simulink model "rotating_pendulum_3states_simulink"  (R2020b)
settings: Solver=FixedStepAuto  StartTime=0.0  StopTime=40  FixedStep=h  RelTol=1e-3  EnableMultiTasking=on
values from neighbouring files (symbols this model uses):
  adingain = [adingain 1 1 1 1 1]    [hwinit.m]
  adinoffs = [adinoffs 0 0 0 0 0]    [hwinit.m]
  daoutgain = 1*[-6]    [hwinit.m]
  daoutoffs = [0.00]    [hwinit.m]
  h = 0.01    [Linearization_4state.m]    (also in hwinit.m = 0.001; rotpentest.m = fugiboard('Open', 'pendulum1'))
  K = model.Km    [Linearization_4state.m]    (also in Model_derivation.m = K_trans + K_rot; Model_derivation_4_states.m = K_trans + K_rot; dc_motor_control.m = dlqr(dt_sys_zoh.A, dt_sys_zoh.B, Q_lqr, R_lqr); identification_dc_motor.m = -0.05)
  K_ff = 1/dcgain_sys    [dc_motor_control.m]    (also in rotating_pendulum_3states.m; rotating_pendulum_4states.m)
  R_kf = 1 * diag([1, 10, 1, 10])    [dc_motor_control.m]    (also in rotating_pendulum_3states.m = 50 * diag([1, 1, 10]); rotating_pendulum_4states.m = diag([7.5740e-06, 0.1526, 1.4489e-05, 0.2930]))
undefined symbols (not defined in the file or in its folder): Discrete, Time
libraries: simulink x3, ctrlSharedLib x1
settings Model: Creator=rbabuska  LastModifiedBy=dlooman
settings DataIOCC: LimitDataPoints=on  SaveFormat=Array  ReturnWorkspaceOutputs=off  SignalLoggingName=sigsOut
settings OptimizationCC: BooleanDataType=off  ExpressionDepthLimit=2147483647  InitFltsAndDblsToZero=on  LifeSpan=inf
settings DebuggingCC: SaveWithParameterizedLinksMsg=none  SignalResolutionControl=TryResolveAllWithWarning  MultiTaskDSMMsg=warning  MultiTaskCondExecSysMsg=none  AllowSymbolicDim=off  StateNameClashWarn=warning  SFUnexpectedBacktrackingDiag=warning  SFNoUnconditionalDefaultTransitionDiag=warning  SFExecutionAtInitializationDiag=none  ArithmeticOperatorsInVariantConditions=warning
settings HardwareCC: ProdBitPerPointer=32  ProdBitPerSizeT=32  ProdBitPerPtrDiffT=32  ProdLargestAtomicFloat=None  ProdIntDivRoundTo=Undefined  ProdEndianess=Unspecified  ProdWordSize=32  ProdHWDeviceType=32-bit Generic  TargetUnknown=on
settings ModelReferenceCC: PropagateSignalLabelsOutOfModel=off
settings SFSimCC: SimUseLocalCustomCode=off  CustomCodeUndefinedFunction=UseInterfaceOnly
settings RTWCC: RTWUseLocalCustomCode=off
settings CodeAppCC: StateflowObjectComments=on
settings GRTTargetCC: TargetFcnLib=ansi_tfl_tmw.mat  TargetLangStandard=C89/C90 (ANSI)  CombineOutputUpdateFcns=off  GRTInterface=on
settings ConfigComp: CovMetricSettings=dw  CovSaveCumulativeToWorkspaceVar=on  CovSaveSingleToWorkspaceVar=on  CovExternalEMLEnable=off

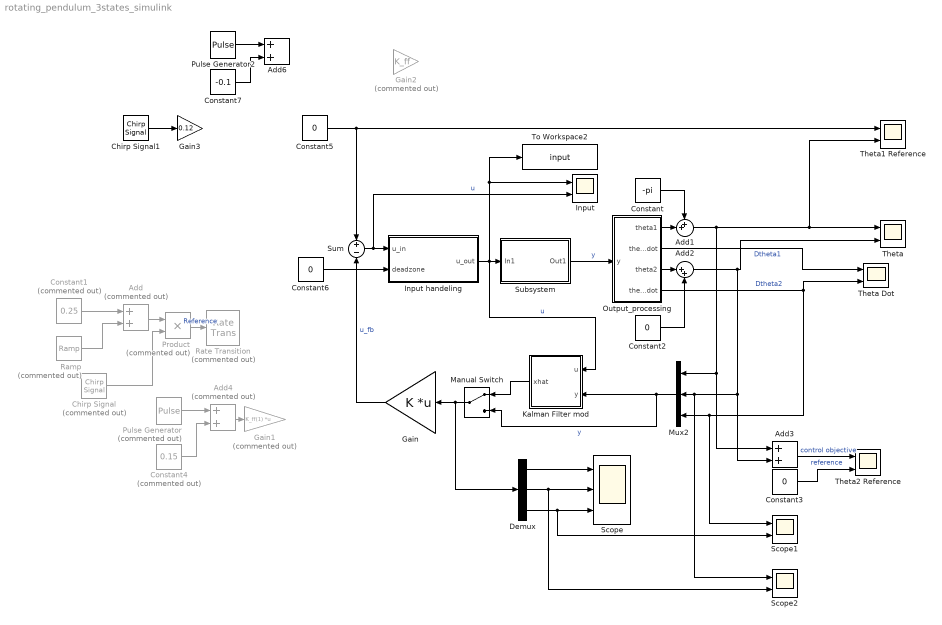
== system rotating_pendulum_3states_simulink ==
  Add : Sum  Commented=on
  Add1 : Sum  Inputs=++|
  Add2 : Sum  Inputs=|++
  Add3 : Sum
  Add4 : Sum  Commented=on
  Add6 : Sum
  Chirp Signal : simulink/Sources/Chirp Signal  Commented=on  f1=3  T=20  f2=1
  Chirp Signal1 : simulink/Sources/Chirp Signal  f1=0.1  T=20  f2=2.5
  Constant : Constant  Value=-pi
  Constant1 : Constant  Commented=on  Value=0.25  SampleTime=h
  Constant{2..3,5..6} (4 alike) : Constant  Value=0
  Constant4 : Constant  Commented=on  Value=0.15
  Constant7 : Constant  Value=-0.1
  Demux : Demux  Outputs=3
  Gain : Gain  Gain=K  Multiplication=Matrix(K*u)
  Gain1 : Gain  Commented=on  Gain=K_ff(1)  Multiplication=Matrix(K*u)
  Gain2 : Gain  Commented=on  Gain=K_ff
  Gain3 : Gain  Gain=0.12
  Input : Scope  NumInputPorts=2
  Input handeling : MATLAB Function  TreatAsAtomicUnit=on
  Kalman Filter mod : Subsystem
  Manual Switch : ManualSwitch
  Mux2 : Mux  Inputs=3
  Output_processing : Subsystem
  Product : Product  Commented=on
  Pulse Generator : DiscretePulseGenerator  Commented=on  PulseType=Time based  Amplitude=-0.3  PulseWidth=50
  Pulse Generator2 : DiscretePulseGenerator  PulseType=Time based  Amplitude=.2  Period=4  PulseWidth=50
  Ramp : simulink/Sources/Ramp  Commented=on  slope=-1/100  start=0  InitialOutput=0
  Rate Transition : RateTransition  Commented=on
  Scope : Scope  NumInputPorts=3
  Scope1 : Scope  NumInputPorts=2
  Scope2 : Scope  NumInputPorts=2
  Subsystem : Subsystem
      mask Display: disp('Rotational\nPendulum')
  Sum : Sum  Inputs=+|-
  Theta : Scope  NumInputPorts=2
  Theta Dot : Scope  NumInputPorts=2
  Theta1 Reference : Scope  NumInputPorts=2
  Theta2 Reference : Scope  NumInputPorts=2
  To Workspace2 : ToWorkspace  VariableName=input  SaveFormat=Timeseries  SampleTime=-1
  wires:
  Sum/1 -> Input/2, Input handeling/1(u_in)  "u"
  Subsystem/1(Out1) -> Output_processing/1(y)  "y"
  Output_processing/2(theta1_dot) -> Theta Dot/1  "Dtheta1"
  Output_processing/3(theta2) -> Add2/1
  Output_processing/4(theta2_dot) -> Theta Dot/2, Mux2/3, Scope1/1  "Dtheta2"
  Product/1 -> Rate Transition/1  "Reference"
  Constant1/1 -> Add/1
  Ramp/1 -> Add/2
  Mux2/1 -> Manual Switch/2, Kalman Filter mod/2(y)  "y"
  Output_processing/1(theta1) -> Add1/2
  Add1/1 -> Theta1 Reference/2, Theta/1, Add3/1, Mux2/1
  Constant/1 -> Add1/1
  Add2/1 -> Theta/2, Scope2/1, Mux2/2, Add3/2
  Constant2/1 -> Add2/2
  Add3/1 -> Theta2 Reference/1  "control objective"
  Add4/1 -> Gain1/1
  Pulse Generator/1 -> Add4/1
  Constant4/1 -> Add4/2
  Add/1 -> Product/1
  Chirp Signal/1 -> Product/2
  Demux/1 -> Scope/1
  Demux/2 -> Scope2/2, Scope/2
  Demux/3 -> Scope1/2, Scope/3
  Chirp Signal1/1 -> Gain3/1
  Constant5/1 -> Sum/1, Theta1 Reference/1
  Manual Switch/1 -> Gain/1, Demux/1
  Kalman Filter mod/1(xhat) -> Manual Switch/1
  Input handeling/1(u_out) -> Input/1, To Workspace2/1, Subsystem/1(In1), Kalman Filter mod/1(u)  "u"
  Constant6/1 -> Input handeling/2(deadzone)
  Gain/1 -> Sum/2  "u_fb"
  Constant7/1 -> Add6/2
  Pulse Generator2/1 -> Add6/1
  Constant3/1 -> Theta2 Reference/2  "reference"

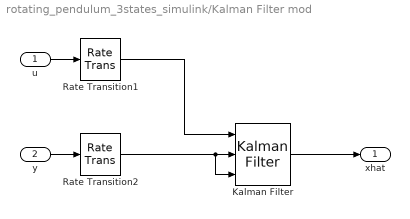
== system rotating_pendulum_3states_simulink/Kalman Filter mod ==
  u : Inport
  y : Inport  Port=2
  Kalman Filter : ctrlSharedLib/Kalman Filter  TimeDomain=Discrete-Time  UseCurrentEstimator=on  ModelSource=LTI State-Space Variable  ModelSourceVariable=dt_sys_zoh  A=0.95  B=1  C=1  D=0  NumberOfStates=1  NumberOfInputs=1  NumberOfOutputs=1  InitialEstimateSource=Input port  X0=[0, 0, 0, 0]  P0=10  UseK=off  UseGH=off  NumberOfProcessNoiseInputs=1  G=1  TimeInvariantG=on  H=0  TimeInvariantH=on  Q=Q_kf  TimeInvariantQ=on  R=R_kf  TimeInvariantR=on  N=0  TimeInvariantN=on  AddInputPort=on  AddEnablePort=off  OutputEstimatedY=off  OutputP=off  Ts=-1
  Rate Transition1 : RateTransition
  Rate Transition2 : RateTransition
  xhat : Outport
  wires:
  Rate Transition2/1 -> Kalman Filter/3, Kalman Filter/2
  Rate Transition1/1 -> Kalman Filter/1
  u/1 -> Rate Transition1/1
  Kalman Filter/1 -> xhat/1
  y/1 -> Rate Transition2/1

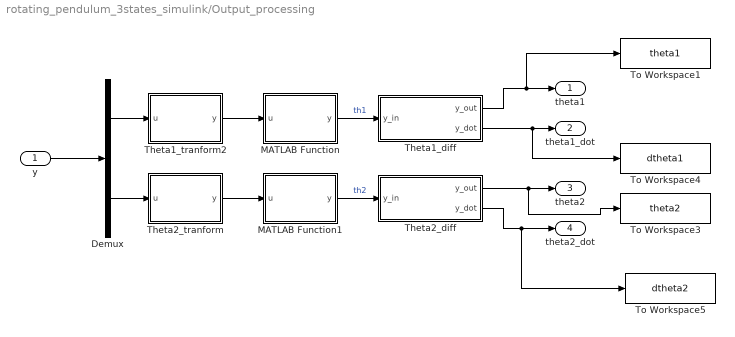
== system rotating_pendulum_3states_simulink/Output_processing ==
  y : Inport
  Demux : Demux  Outputs=2
  MATLAB Function : MATLAB Function  TreatAsAtomicUnit=on
  MATLAB Function1 : MATLAB Function  TreatAsAtomicUnit=on
  Theta1_diff : Subsystem
  Theta1_tranform2 : MATLAB Function  TreatAsAtomicUnit=on
  Theta2_diff : Subsystem
  Theta2_tranform : MATLAB Function  TreatAsAtomicUnit=on
  To Workspace1 : ToWorkspace  VariableName=theta1  SaveFormat=Timeseries  SampleTime=-1
  To Workspace3 : ToWorkspace  VariableName=theta2  SaveFormat=Timeseries  SampleTime=-1
  To Workspace4 : ToWorkspace  VariableName=dtheta1  SaveFormat=Timeseries  SampleTime=-1
  To Workspace5 : ToWorkspace  VariableName=dtheta2  SaveFormat=Timeseries  SampleTime=-1
  theta1 : Outport
  theta1_dot : Outport  Port=2
  theta2 : Outport  Port=3
  theta2_dot : Outport  Port=4
  wires:
  y/1 -> Demux/1
  Theta2_diff/1(y_out) -> To Workspace3/1, theta2/1
  Theta1_diff/2(y_dot) -> To Workspace4/1, theta1_dot/1
  Demux/1 -> Theta1_tranform2/1(u)
  Demux/2 -> Theta2_tranform/1(u)
  Theta2_diff/2(y_dot) -> To Workspace5/1, theta2_dot/1
  Theta1_diff/1(y_out) -> To Workspace1/1, theta1/1
  Theta1_tranform2/1(y) -> MATLAB Function/1(u)
  MATLAB Function/1(y) -> Theta1_diff/1(y_in)  "th1"
  MATLAB Function1/1(y) -> Theta2_diff/1(y_in)  "th2"
  Theta2_tranform/1(y) -> MATLAB Function1/1(u)

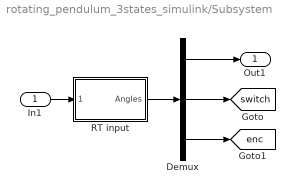
== system rotating_pendulum_3states_simulink/Subsystem ==
  In1 : Inport
  Demux : Demux  Outputs=[2 4 1]
  RT input : Subsystem  mask{Ts=h, channels=[6 7]}
      mask prompts: Ts "Sample time [s]:"; channels "Channels to read (e.g., [6 7])"
      mask init:
      | hwinit;
      | 
      | % initialize FPGA
      | fugihandle = fugiboard('Open', 'Pendulum1');
      | fugihandle.WatchdogTimeout = 0.5;
      | fugiboard('SetParams', fugihandle);
      | fugiboard('Write', fugihandle, 0, 0, 0, 0);  % dummy write to sync interface board
      | fugiboard('Write', fugihandle, 5, 1, 0, 0);  % reset position, activate relay
      | data = fugiboard('Read', fugihandle);        % get version info from FPGA
      | % model = bitshift(data(1), -5); 
      | % version = bitand(data(1), 31);
      | % disp(sprintf('FPGA setup %d, version %d', model, version)); % for the B&P it should say 1 1, or else there is a problem
      | fugiboard('Write', fugihandle, 0, 1, 0, 0);  % end reset
      | pause(0.1);                         % give relay some time to respond
      mask Display: disp('Rotational\nPendulum')
  Out1 : Outport
  tag scope: enc=global, switch=global
  wires:
  RT input/1(Angles) -> Demux/1
  Demux/1 -> Out1/1
  Demux/2 -> [switch]
  Demux/3 -> [enc]
  In1/1 -> RT input/1(Motors)

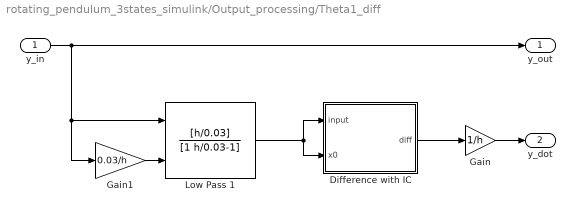
== system rotating_pendulum_3states_simulink/Output_processing/Theta1_diff ==
  y_in : Inport
  Difference with IC : Subsystem
  Gain : Gain  Gain=1/h
  Gain1 : Gain  Gain=0.03/h
  Low Pass 1 : DiscreteTransferFcn  Numerator=[h/0.03]  Denominator=[1 h/0.03-1]  InitialStatesSource=Input port
      settings: InputPortMap=u0,p5
  y_out : Outport
  y_dot : Outport  Port=2
  wires:
  y_in/1 -> y_out/1, Gain1/1, Low Pass 1/1
  Low Pass 1/1 -> Difference with IC/1(input), Difference with IC/2(x0)
  Gain/1 -> y_dot/1
  Gain1/1 -> Low Pass 1/2
  Difference with IC/1(diff) -> Gain/1

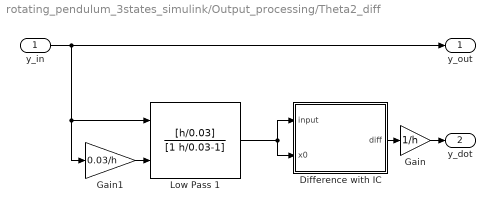
== system rotating_pendulum_3states_simulink/Output_processing/Theta2_diff ==
  y_in : Inport
  Difference with IC : Subsystem
  Gain : Gain  Gain=1/h
  Gain1 : Gain  Gain=0.03/h
  Low Pass 1 : DiscreteTransferFcn  Numerator=[h/0.03]  Denominator=[1 h/0.03-1]  InitialStatesSource=Input port
      settings: InputPortMap=u0,p5
  y_out : Outport
  y_dot : Outport  Port=2
  wires:
  y_in/1 -> y_out/1, Gain1/1, Low Pass 1/1
  Difference with IC/1(diff) -> Gain/1
  Low Pass 1/1 -> Difference with IC/2(x0), Difference with IC/1(input)
  Gain/1 -> y_dot/1
  Gain1/1 -> Low Pass 1/2

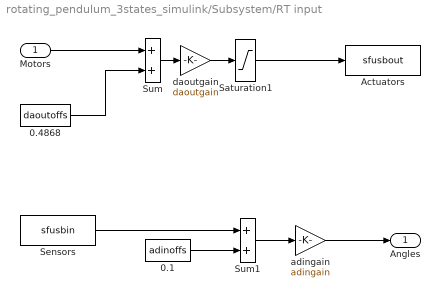
== system rotating_pendulum_3states_simulink/Subsystem/RT input ==
  Motors : Inport
  0.1 : Constant  Value=adinoffs
  0.4868 : Constant  Value=daoutoffs
  Actuators : S-Function  FunctionName=sfusbout  Parameters=Ts, fugihandle  SFunctionDeploymentMode=off  EnableBusSupport=off
  Saturation1 : Saturate  UpperLimit=10  LowerLimit=-10
  Sensors : S-Function  FunctionName=sfusbin  Parameters=Ts, fugihandle, channels  SFunctionDeploymentMode=off  EnableBusSupport=off
  Sum : Sum  InputSameDT=on  SaturateOnIntegerOverflow=on  OutDataTypeStr=Inherit: Same as first input
  Sum1 : Sum  InputSameDT=on  SaturateOnIntegerOverflow=on  OutDataTypeStr=Inherit: Same as first input
  adingain : Gain  Gain=adingain  SaturateOnIntegerOverflow=on  OutDataTypeStr=Inherit: Same as input  ParamDataTypeStr=Inherit: Same as input
  daoutgain : Gain  Gain=daoutgain  SaturateOnIntegerOverflow=on  OutDataTypeStr=Inherit: Same as input  ParamDataTypeStr=Inherit: Same as input
  Angles : Outport
  wires:
  Sum/1 -> daoutgain/1
  0.4868/1 -> Sum/2
  Motors/1 -> Sum/1
  Sum1/1 -> adingain/1
  0.1/1 -> Sum1/2
  adingain/1 -> Angles/1
  Saturation1/1 -> Actuators/1
  daoutgain/1 -> Saturation1/1
  Sensors/1 -> Sum1/1

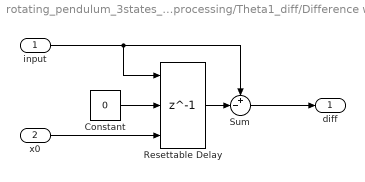
== system rotating_pendulum_3states_simulink/Output_processing/Theta1_diff/Difference with IC ==
  input : Inport
  x0 : Inport  Port=2
  Constant : Constant  Value=0
  Resettable Delay : Delay  DelayLength=1  InitialConditionSource=Input port  ExternalReset=Rising
      settings: InputPortMap=u0,r5,p4
  Sum : Sum  Inputs=+-|
  diff : Outport
  wires:
  input/1 -> Resettable Delay/1, Sum/1
  Constant/1 -> Resettable Delay/2
  Sum/1 -> diff/1
  Resettable Delay/1 -> Sum/2
  x0/1 -> Resettable Delay/3

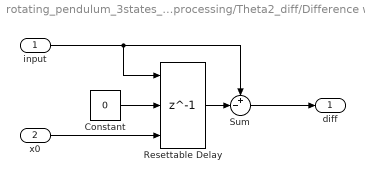
== system rotating_pendulum_3states_simulink/Output_processing/Theta2_diff/Difference with IC ==
  input : Inport
  x0 : Inport  Port=2
  Constant : Constant  Value=0
  Resettable Delay : Delay  DelayLength=1  InitialConditionSource=Input port  ExternalReset=Rising
      settings: InputPortMap=u0,r5,p4
  Sum : Sum  Inputs=+-|
  diff : Outport
  wires:
  input/1 -> Resettable Delay/1, Sum/1
  Constant/1 -> Resettable Delay/2
  Sum/1 -> diff/1
  Resettable Delay/1 -> Sum/2
  x0/1 -> Resettable Delay/3

== matlab function rotating_pendulum_3states_simulink/Output_processing/Theta1_tranform2 ==
  data: u input; y output
function y = fcn2(u)
if (u<0)
    u = u+2*pi;
end
y = u;

== matlab function rotating_pendulum_3states_simulink/Output_processing/MATLAB Function1 ==
  data: u input; y output
function y = conv_online(u)
persistent corr prev
        
if isempty(corr)
    corr = 0;
    prev = 0;
end

if u-prev > 5.8
    corr = corr - 2*pi;
elseif u-prev < -5.8
    corr = corr + 2*pi;
end

prev=u;
y=u+corr;
end

== matlab function rotating_pendulum_3states_simulink/Output_processing/Theta2_tranform ==
  data: u input; y output
function y = fcn(u)
if (u<0)
    u = u+2*pi;
end
u=u-pi;
y = u;

== matlab function rotating_pendulum_3states_simulink/Input handeling ==
  data: u_in input; u_out output; deadzone input
function u_out = fcn(u_in, deadzone)
% input handeling: deadzone compensation and saturation
max_u = 1; % Do Not change
gain = (max_u - deadzone);

if u_in > 0.2*deadzone
    u_out = gain * u_in + deadzone;
elseif u_in < -0.2*deadzone
    u_out = gain * u_in - deadzone;
else
    u_out = 0;
end

% Saturation handeling
if u_out > max_u
    u_out = max_u;
elseif u_out < -max_u
    u_out = -max_u;
end

== matlab function rotating_pendulum_3states_simulink/Output_processing/MATLAB Function ==
  data: u input; y output
function y = conv_online(u)
persistent corr prev
        
if isempty(corr)
    corr = 0;
    prev = 0;
end

if u-prev > 5.8
    corr = corr - 2*pi;
elseif u-prev < -5.8
    corr = corr + 2*pi;
end

prev=u;
y=u+corr;
end
